simulink model "Farmakodynamika_22a"  (R2022a)
settings: Solver=VariableStepAuto  StartTime=0.0  StopTime=600  FixedStep=1  RelTol=1e-3
values from neighbouring files (symbols this model uses):
  Gb = 153    [params.m]
  ki = Pop(i,3)    [fitness.m]    (also in gen3.m = best_ch(3,end); params.m = 0.1629)
  p2 = Pop(i,1)    [fitness_dk.m]    (also in params.m = best_ch(1,end))
  Sg = 0    [params.m]
  Si = Pop(i,2)    [fitness_dk.m]    (also in params.m = best_ch(2,end))
  Ti = Pop(i,1)    [fitness.m]    (also in gen3.m = best_ch(1,end); params.m = 45.383)
  v = 281.218    [fitness.m]    (also in fitness_dk.m; gen3.m = 281.28; params.m = 281.28)
  Vg = 1.467    [params.m]
  Vi = Pop(i,2)    [fitness.m]    (also in gen3.m = best_ch(2,end); params.m = 139.094)
  weight = 64.4    [params.m]
settings Model: Creator=DFUNDO  LastModifiedBy=DFUNDO
settings ModelReferenceCC: EnableRefExpFcnMdlSchedulingChecks=off
settings RTWCC: Description=Generic Real-Time Target

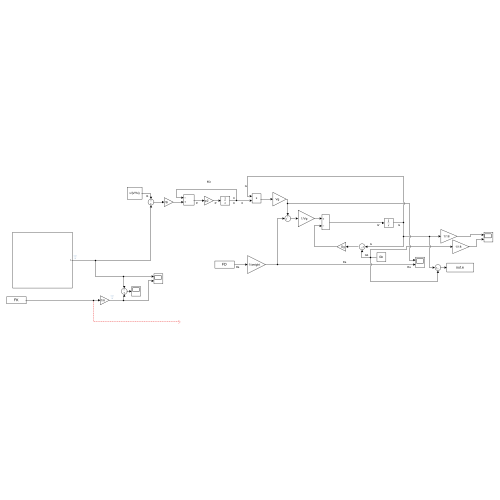
[thumbnail: Simulink's stored preview of the top-level diagram]
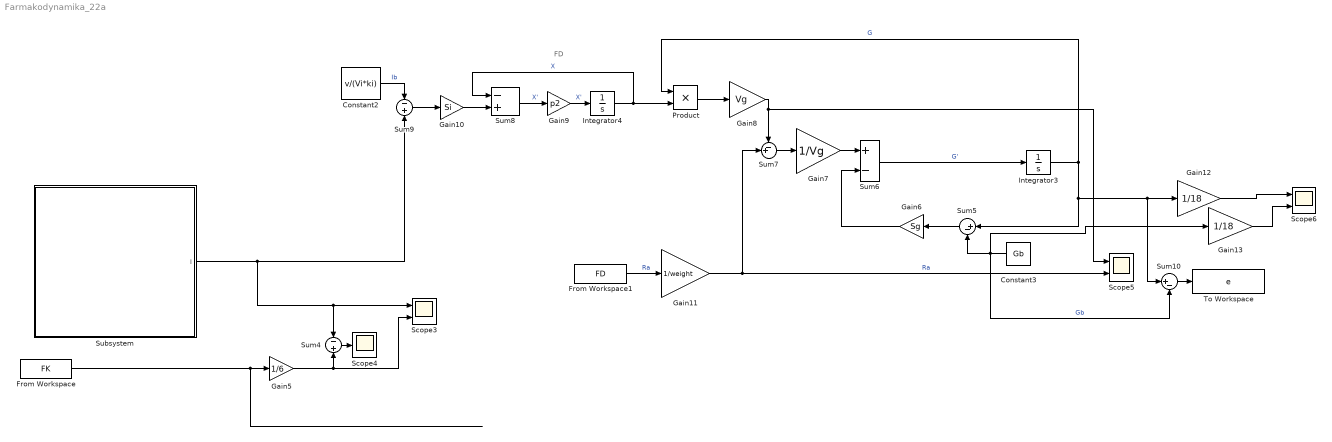
== system Farmakodynamika_22a ==
  note: FD
  Constant2 : Constant  Value=v/(Vi*ki)
  Constant3 : Constant  Value=Gb
  From Workspace : FromWorkspace  VariableName=FK
  From Workspace1 : FromWorkspace  VariableName=FD
  Gain10 : Gain  Gain=Si
  Gain11 : Gain  Gain=1/weight
  Gain12 : Gain  Gain=1/18
  Gain13 : Gain  Gain=1/18
  Gain5 : Gain  Gain=1/6
  Gain6 : Gain  Gain=Sg
  Gain7 : Gain  Gain=1/Vg
  Gain8 : Gain  Gain=Vg
  Gain9 : Gain  Gain=p2
  Integrator3 : Integrator  InitialCondition=Gb
  Integrator4 : Integrator
  Product : Product
  Scope3 : Scope  NumInputPorts=2
  Scope4 : Scope
  Scope5 : Scope  NumInputPorts=2
  Scope6 : Scope  NumInputPorts=2
  Subsystem : Subsystem
  Sum10 : Sum  Inputs=|+-
  Sum4 : Sum  Inputs=-+
  Sum5 : Sum  Inputs=|+-
  Sum6 : Sum  Inputs=+-
  Sum7 : Sum  Inputs=-+|
  Sum8 : Sum  Inputs=-+
  Sum9 : Sum  Inputs=-+
  To Workspace : ToWorkspace  VariableName=e  SampleTime=-1
      settings: Save2DSignal=2-D array (concatenate along first dimension)
  wires:
  From Workspace/1 -> Gain5/1
  Sum4/1 -> Scope4/1
  Gain5/1 -> Sum4/2, Scope3/2
  Integrator3/1 -> Product/1, Sum5/1, Sum10/1, Gain12/1  "G"
  Sum6/1 -> Integrator3/1  "G'"
  Sum5/1 -> Gain6/1
  Constant3/1 -> Gain13/1, Sum5/2, Sum10/2  "Gb"
  Gain6/1 -> Sum6/2
  Product/1 -> Gain8/1
  Sum7/1 -> Gain7/1
  Gain8/1 -> Scope5/1, Sum7/1
  Gain7/1 -> Sum6/1
  Integrator4/1 -> Product/2, Sum8/1  "X"
  Gain9/1 -> Integrator4/1  "X'"
  Sum8/1 -> Gain9/1  "X'"
  Gain10/1 -> Sum8/2
  Constant2/1 -> Sum9/1  "Ib"
  Sum9/1 -> Gain10/1
  Gain11/1 -> Sum7/2, Scope5/2  "Ra"
  From Workspace1/1 -> Gain11/1  "Ra"
  Sum10/1 -> To Workspace/1
  Gain12/1 -> Scope6/1
  Gain13/1 -> Scope6/2
  Subsystem/1(I) -> Sum9/2, Sum4/1, Scope3/1

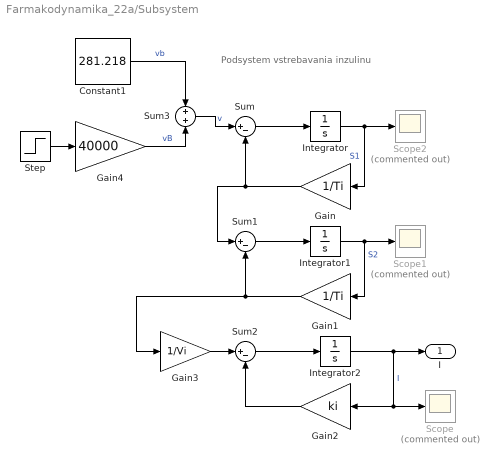
== system Farmakodynamika_22a/Subsystem ==
  note: Podsystem vstrebavania inzulinu
  Constant1 : Constant  Value=281.218
  Gain : Gain  Gain=1/Ti
  Gain1 : Gain  Gain=1/Ti
  Gain2 : Gain  Gain=ki
  Gain3 : Gain  Gain=1/Vi
  Gain4 : Gain  Gain=40000
  Integrator : Integrator  InitialCondition=Ti*v
  Integrator1 : Integrator  InitialCondition=Ti*v
  Integrator2 : Integrator  InitialCondition=v/(Vi*ki)
  Scope : Scope  Commented=on
  Scope1 : Scope  Commented=on
  Scope2 : Scope  Commented=on
  Step : Step  Time=5  Before=1  After=0  SampleTime=0
  Sum : Sum  Inputs=|+-
  Sum1 : Sum  Inputs=|+-
  Sum2 : Sum  Inputs=|+-
  Sum3 : Sum
  I : Outport
  wires:
  Gain2/1 -> Sum2/2
  Integrator1/1 -> Scope1/1, Gain1/1  "S2"
  Gain/1 -> Sum/2, Sum1/1
  Sum2/1 -> Integrator2/1
  Sum1/1 -> Integrator1/1
  Sum3/1 -> Sum/1  "v"
  Integrator/1 -> Gain/1, Scope2/1  "S1"
  Gain1/1 -> Gain3/1, Sum1/2
  Gain3/1 -> Sum2/1
  Constant1/1 -> Sum3/1  "vb"
  Integrator2/1 -> Gain2/1, Scope/1, I/1  "I"
  Sum/1 -> Integrator/1
  Step/1 -> Gain4/1
  Gain4/1 -> Sum3/2  "vB"
